simulink library "State_Machine"  (R2015a)
settings: Solver=ode45  SolverMode=SingleTasking  StartTime=0.0  StopTime=10.0  RelTol=1e-3
undefined symbols (not defined in the file): THETA_BALANCING, THETA_SWING, THETA_WAIT, TORQUE_LEVEL
libraries: State_Machine x1
settings Model: Creator=sdupertu  LastModifiedBy=sdupertu
settings OptimizationCC: BlockReduction=off  BooleanDataType=off
settings DebuggingCC: SaveWithParameterizedLinksMsg=none  UnderspecifiedInitializationDetection=Classic  MergeDetectMultiDrivingBlocksExec=none  SignalResolutionControl=TryResolveAllWithWarning  StrictBusMsg=Warning
settings HardwareCC: TargetUnknown=on

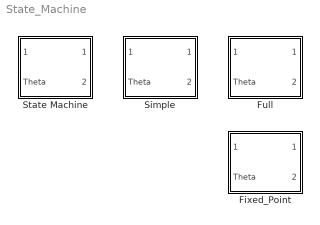
== system State_Machine ==
  Fixed_Point : Subsystem
  Full : Subsystem
  Simple : Subsystem
  State Machine : Subsystem  BlockChoice=Full
      settings: TemplateBlock=self  MemberBlocks=Fixed_Point,Full,Simple
      mask Display: image('State_Machine_Diagram.png');

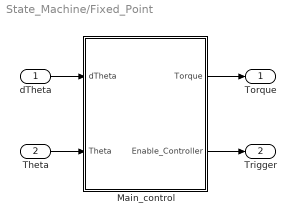
== system State_Machine/Fixed_Point ==
  dTheta : Inport
  Theta : Inport  Port=2
  Main_control : Stateflow chart  TreatAsAtomicUnit=on
  Torque : Outport
  Trigger : Outport  Port=2
  wires:
  Main_control/2(Enable_Controller) -> Trigger/1
  Main_control/1(Torque) -> Torque/1
  dTheta/1 -> Main_control/1(dTheta)
  Theta/1 -> Main_control/2(Theta)

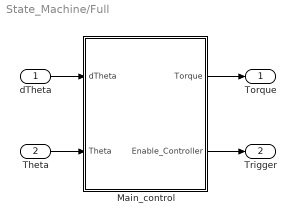
== system State_Machine/Full ==
  dTheta : Inport
  Theta : Inport  Port=2
  Main_control : Stateflow chart  TreatAsAtomicUnit=on
  Torque : Outport
  Trigger : Outport  Port=2
  wires:
  Main_control/2(Enable_Controller) -> Trigger/1
  Main_control/1(Torque) -> Torque/1
  dTheta/1 -> Main_control/1(dTheta)
  Theta/1 -> Main_control/2(Theta)

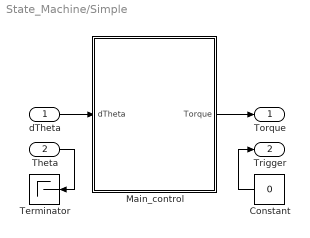
== system State_Machine/Simple ==
  dTheta : Inport
  Theta : Inport  Port=2
  Constant : Constant  Value=0
  Main_control : Stateflow chart  TreatAsAtomicUnit=on
  Terminator : Terminator
  Torque : Outport
  Trigger : Outport  Port=2
  wires:
  Theta/1 -> Terminator/1
  dTheta/1 -> Main_control/1(dTheta)
  Main_control/1(Torque) -> Torque/1
  Constant/1 -> Trigger/1

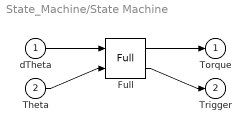
== system State_Machine/State Machine ==
  dTheta : Inport
  Theta : Inport  Port=2
  Full : State_Machine/Full  SystemSampleTime=-1
  Torque : Outport
  Trigger : Outport  Port=2
  wires:
  dTheta/1 -> Full/1
  Theta/1 -> Full/2
  Full/1 -> Torque/1
  Full/2 -> Trigger/1

== stateflow chart State_Machine/Full/Main_control ==
  settings: executeAtInitialization=1
  state Startup
  state Swingright
    during:
    Torque = TORQUE_LEVEL;
  state Swingleft
    during:
    Torque = -TORQUE_LEVEL;
  state Wait
    entry:
    Torque = 0;
  state Balancing
    entry:
    Enable_Controller = 1;
    exit:
    Enable_Controller = 0;
  (default) -> Startup : {Enable_Controller = 0; Torque = 0;}
  (junction 27) -> Startup
  Startup -> (junction 7) [order 1] : [dTheta > 0]
  (junction 28) -> (junction 27)
  (junction 7) -> Swingright
  Startup -> Swingleft [order 2]
  Swingleft -> Swingright [order 2] : [dTheta > 0]
  Swingright -> Swingleft [order 2] : [dTheta < 0]
  Swingright -> Wait [order 1] : [Theta < THETA_WAIT]
  Swingleft -> Wait [order 1] : [Theta < THETA_WAIT]
  Wait -> (junction 28) [order 2] : [Theta > THETA_SWING]
  (junction 33) -> (junction 28)
  Wait -> Balancing [order 1] : [Theta < THETA_BALANCING]
  Balancing -> (junction 33) : [Theta > THETA_SWING]
  data: dTheta input double; Torque output double; Enable_Controller output boolean; Theta input double; THETA_BALANCING parameter; THETA_SWING parameter; THETA_WAIT parameter; TORQUE_LEVEL parameter

== stateflow chart State_Machine/Simple/Main_control ==
  state Startup
  state Swingleft
    during:
    Torque = -TORQUE_LEVEL;
  state Swingright
    during:
    Torque = TORQUE_LEVEL;
  (default) -> Startup : {Torque = 0;}
  Startup -> (junction 7) [order 1] : [dTheta > 0]
  (junction 7) -> Swingright
  Startup -> Swingleft [order 2]
  Swingleft -> Swingright : [dTheta > 0]
  Swingright -> Swingleft : [dTheta < 0]
  data: dTheta input double; Torque output double; TORQUE_LEVEL parameter

== stateflow chart State_Machine/Fixed_Point/Main_control ==
  settings: executeAtInitialization=1
  state Startup
  state Swingright
    during:
    Torque = TORQUE_LEVEL;
  state Swingleft
    during:
    Torque = -TORQUE_LEVEL;
  state Wait
    entry:
    Torque = 0;
  state Balancing
    entry:
    Enable_Controller = 1;
    exit:
    Enable_Controller = 0;
  (default) -> Startup : {Enable_Controller = 0; Torque = 0;}
  (junction 27) -> Startup
  Startup -> (junction 7) [order 1] : [dTheta > 0]
  (junction 28) -> (junction 27)
  (junction 7) -> Swingright
  Startup -> Swingleft [order 2]
  Swingleft -> Swingright [order 2] : [dTheta > 0]
  Swingright -> Swingleft [order 2] : [dTheta < 0]
  Swingright -> Wait [order 1] : [Theta < THETA_WAIT]
  Swingleft -> Wait [order 1] : [Theta < THETA_WAIT]
  Wait -> (junction 28) [order 2] : [Theta > THETA_SWING]
  (junction 33) -> (junction 28)
  Wait -> Balancing [order 1] : [Theta < THETA_BALANCING]
  Balancing -> (junction 33) : [Theta > THETA_SWING]
  data: dTheta input fixdt(1,16,7); Torque output fixdt(1,16,7); Enable_Controller output boolean; Theta input fixdt(1,16,7); THETA_BALANCING parameter fixdt(1,16,7); THETA_SWING parameter fixdt(1,16,7); THETA_WAIT parameter fixdt(1,16,7); TORQUE_LEVEL parameter fixdt(1,16,7)
